simulink model "stanley_model"  (R2022a)
settings: Solver=FixedStepAuto  StartTime=0.0  StopTime=Ts  FixedStep=sampling  RelTol=1e-3
values from neighbouring files (symbols this model uses):
  curvature = (DX.*D2Y - DY.*D2X) ./(DX.^2+DY.^2).^(3/2)    [initiateHybrid.m]
  direction = ones(length(gradbp),1)    [initiateHybrid.m]
  gradbp = linspace(0,totalDistance,50)    [initiateHybrid.m]
  L = 3    [MultiAgent_initiateSAC.m]    (also in control_velocity.m; initiate.m; initiateHybrid.m; initiateSAC.m)
  ld = 5    [MultiAgent_initiateSAC.m]    (also in control_velocity.m; initiate.m; initiateHybrid.m; initiateSAC.m)
  psi_o = 0    [MultiAgent_initiateSAC.m]    (also in control_velocity.m; initiate.m; initiateHybrid.m = thetaRefs(1)*(pi/180); initiateSAC.m)
  thetaRefs = smooth(gradbp,thetaRef)    [initiateHybrid.m]
  vel = 5    [MultiAgent_initiateSAC.m]    (also in control_velocity.m = 7; initiate.m = 10; initiateHybrid.m; initiateSAC.m)
  X_o = refPose(1,1)+0    [MultiAgent_initiateSAC.m]    (also in control_velocity.m; initiate.m = refPose(1,1)+60; initiateHybrid.m = xRef(1); initiateSAC.m)
  xRef = refPose(:,1)    [MultiAgent_initiateSAC.m]    (also in control_velocity.m; initiate.m; initiateHybrid.m; initiateSAC.m)
  xRef2s = smooth(gradbp,xRef2)    [initiateHybrid.m]
  xteInt = sqrt((cnormal_xRef(idxc(1))-X_o)^2+(cnormal_yRef(idxc(1))-Y_o)^2)    [MultiAgent_initiateSAC.m]    (also in control_velocity.m; initiate.m; initiateSAC.m; initiateTD3.m)
  Y_o = -refPose(1,2)+20    [MultiAgent_initiateSAC.m]    (also in control_velocity.m = -refPose(1,2)+0; initiate.m; initiateHybrid.m = yRef(1); initiateSAC.m = -refPose(1,2)+0)
  yRef = -refPose(:,2)    [MultiAgent_initiateSAC.m]    (also in control_velocity.m; initiate.m; initiateHybrid.m; initiateSAC.m)
  yRef2s = smooth(gradbp,yRef2)    [initiateHybrid.m]
libraries: simulink_extras x2, simulink x2, vehdynlibviscommon x1, drivingvehiclecontroller x1, robotalgslib x1, autolibshared x1
settings Model: Creator=berka  LastModifiedBy=berka
settings DebuggingCC: UnconnectedInputMsg=warning  UnconnectedOutputMsg=warning  UnconnectedLineMsg=warning
settings RTWCC: DLArmComputeVersion=19.05

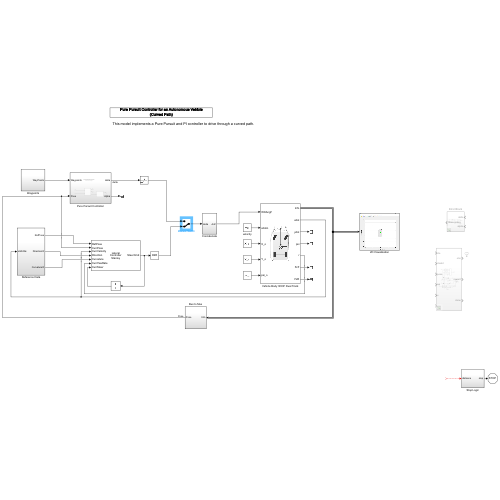
[thumbnail: Simulink's stored preview of the top-level diagram]
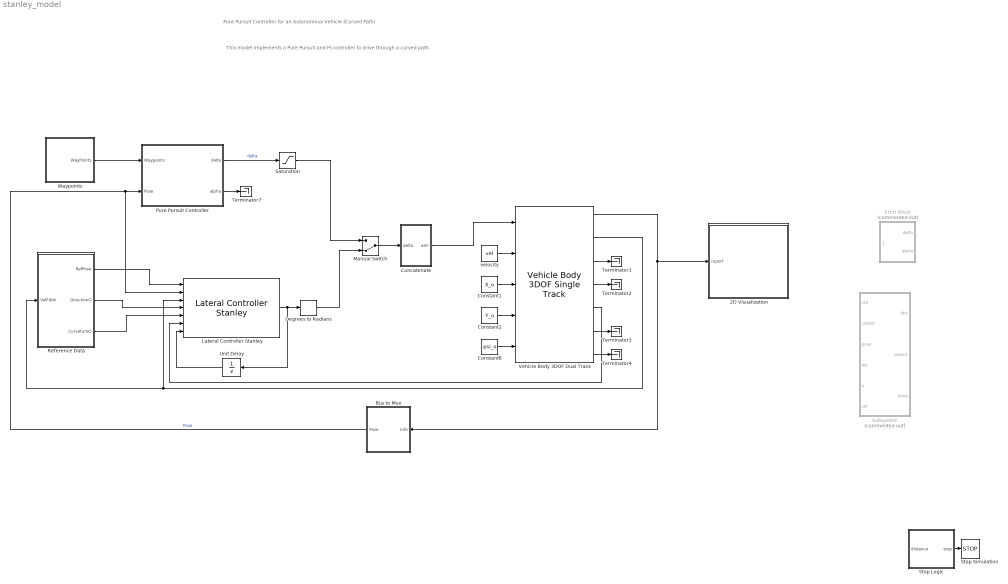
== system stanley_model ==
  note: This model implements a Pure Pursuit and PI controller to drive through a curved path.
  note: Pure Pursuit Controller for an Autonomous Vehicle
      | (Curved Path)
  2D Visualization : Subsystem
      mask Display: image("visualization.JPG");
  Bus to Mux : Subsystem
  Concatenate : Subsystem
  Constant1 : Constant  Value=X_o
  Constant2 : Constant  Value=Y_o
  Constant8 : Constant  Value=psi_o
  Degrees to Radians : simulink_extras/Transformations/Degrees to Radians
  Error Block : Subsystem  Commented=on
  Lateral Controller Stanley : drivingvehiclecontroller/Lateral Controller Stanley  ModelType=Dynamic bicycle model  PositionGainF=2.5  PositionGainR=2.5  YawRateGain=0.2  DelayGain=0.2  VehicleMass=2000  Lf=1.4  Lr=1.6  TireStiffness=12e3  Wheelbase=3  MaxSteeringAngle=35
      settings: SourceProductBaseCode=DR
  Manual Switch : ManualSwitch  CurrentSetting=0
  Pure Pursuit Controller : Subsystem
  Reference Data : Subsystem  VariantControl=Stanley
  Saturation : Saturate
  Stop Logic : Subsystem
  Stop Simulation : Stop
  Subsystem : Subsystem  Commented=on
  Terminator{1..4,7} (5 alike) : Terminator
  Unit Delay : UnitDelay  SampleTime=-1  HasFrameUpgradeWarning=on
  Vehicle Body 3DOF Dual Track : autolibshared/Vehicle Body 3DOF Single Track  trackMode=Dual  inputMode=External longitudinal velocity  frontSteerMode=on  rearSteerMode=off  windMode=off  muMode=off  extFMode=off  extMMode=off  htchFMode=off  htchMMode=off  extXo=on  extpsio=on  extxdoto=off  extro=off  extYo=on  extTamb=off  extydoto=off  aMode=2  NF=2  NR=2  m=2000  a=1.4  b=1.6  h=0.35  dh=1  hh=0.2  X_o=0  xdot_o=0  CalphaMode=off  sigmaMode=on  d=0  hl=0  w=[1.4,1.4]  Cy_f=12e3  Cy_r=11e3  sigma_f=.1  sigma_r=.1  alpha_f_brk=[-.1 .1]  Cy_f_data=[-9e3 9e3]  alpha_r_brk=[-.1 .1]  Cy_r_data=[-9e3 9e3]  Y_o=0  ydot_o=0  Izz=4000  psi_o=0  r_o=0  Af=2  Cd=.3  Cl=.1  Cpm=.1  beta_w=[0:0.01:0.3]  Cs=[0:0.03:0.9]  Cym=[0:0.01:0.3]  Pabs=101325  Tair=273  g=9.81  mu=1  xdot_tol=.01  Fznom=5000  Fxtire_sat=7e4  Fytire_sat=7e4  longOff=0  latOff=0  vertOff=0  wrapAng=off
      settings: SourceProductBaseCode=PW,DR,MT,VE
  Waypoints : Subsystem
  velocity : Constant  Value=vel
  wires:
  Constant1/1 -> Vehicle Body 3DOF Dual Track/3
  Vehicle Body 3DOF Dual Track/3 -> Terminator1/1
  Vehicle Body 3DOF Dual Track/1 -> Bus to Mux/1(Info), 2D Visualization/1(Inport)
  Constant8/1 -> Vehicle Body 3DOF Dual Track/5
  Concatenate/1(AnF) -> Vehicle Body 3DOF Dual Track/1
  Vehicle Body 3DOF Dual Track/6 -> Terminator3/1
  Constant2/1 -> Vehicle Body 3DOF Dual Track/4
  Vehicle Body 3DOF Dual Track/7 -> Terminator4/1
  Vehicle Body 3DOF Dual Track/4 -> Terminator2/1
  Vehicle Body 3DOF Dual Track/5 -> Lateral Controller Stanley/6
  Waypoints/1(WayPoints) -> Pure Pursuit Controller/1(Waypoints)
  Bus to Mux/1(Pose) -> Pure Pursuit Controller/2(Pose), Lateral Controller Stanley/2  "Pose"
  Pure Pursuit Controller/1(delta) -> Saturation/1  "delta"
  velocity/1 -> Vehicle Body 3DOF Dual Track/2
  Reference Data/2(DirectionO) -> Lateral Controller Stanley/4
  Reference Data/3(CurvatureO) -> Lateral Controller Stanley/5
  Reference Data/1(RefPose) -> Lateral Controller Stanley/1
  Lateral Controller Stanley/1 -> Unit Delay/1, Degrees to Radians/1
  Unit Delay/1 -> Lateral Controller Stanley/7
  ? -> Stop Logic/1(distance)
  Stop Logic/1(stop) -> Stop Simulation/1
  Pure Pursuit Controller/2(alpha) -> Terminator7/1
  Manual Switch/1 -> Concatenate/1(delta)
  Saturation/1 -> Manual Switch/1
  Degrees to Radians/1 -> Manual Switch/2
  Vehicle Body 3DOF Dual Track/2 -> Reference Data/1(VelFdbk), Lateral Controller Stanley/3

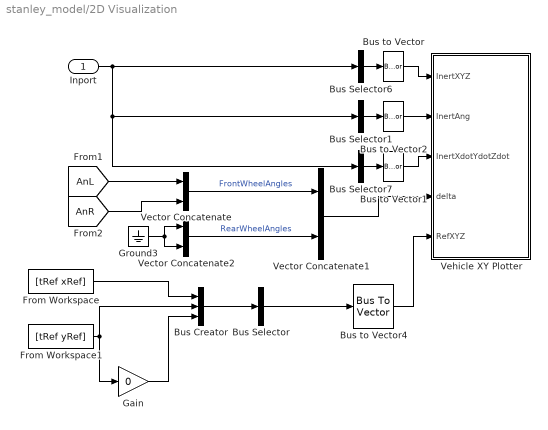
== system stanley_model/2D Visualization ==
  Inport : Inport
  Bus Creator : BusCreator  Inputs=3
  Bus Selector : BusSelector  OutputSignals=signal1,signal2,signal3  OutputAsBus=on
  Bus Selector1 : BusSelector  OutputSignals=InertFrm.Cg.Ang.phi,InertFrm.Cg.Ang.theta,InertFrm.Cg.Ang.psi  OutputAsBus=on
  Bus Selector6 : BusSelector  OutputSignals=InertFrm.Geom.Disp.X,InertFrm.Geom.Disp.Y,InertFrm.Geom.Disp.Z  OutputAsBus=on
  Bus Selector7 : BusSelector  OutputSignals=InertFrm.Geom.Vel.Xdot,InertFrm.Geom.Vel.Ydot,InertFrm.Geom.Vel.Zdot  OutputAsBus=on
  Bus to Vector{,1..2,4} (4 alike) : BusToVector
  From Workspace : FromWorkspace  VariableName=[tRef xRef]
  From Workspace1 : FromWorkspace  VariableName=[tRef yRef]
  Gain : Gain  Gain=0
  Ground3 : Ground
  Vector Concatenate : Concatenate
  Vector Concatenate1 : Concatenate
  Vector Concatenate2 : Concatenate
  Vehicle XY Plotter : Subsystem  mask(Vehicle XY Plotter){a=2, b=2, w=2, figBorder=10, bufferSize=1024, extRef=on, pltDT=.2}
      mask prompts: a "Distance to front axle from CG, a [m]:"; b "Distance to rear axle from CG, b [m]:"; w "Track width, w [m]:"; figBorder "Distance to figure borders, figBorder [m]:"; bufferSize "Path buffer sampe size, bufferSize []:"; extRef "Plot path reference, extRef"; pltDT "Plot update rate, pltDT [s]:"
      mask help:
      | This block will display a MATLAB figure which indicates the vehicle path, current position and heading velocity.
      | An optional path reference is also provided.
      mask init:
      | if autoblkschecksimstopped(gcb)
      |     PortName = 'RefXYZ';
      |     InportOption  = {'built-in/Ground', [PortName, ' Ground'];...
      |         'built-in/Inport',PortName };
      |     if ~strcmp(get_param(gcb,'extRef'),'on')
      |         NewBlkHdl = autoblksreplaceblock(gcb, InportOption, 1);
      |         set_param(NewBlkHdl, 'ShowName', 'off');
      |     else
      |         autoblksreplaceblock(gcb, InportOption, 2);
      |     end
      | end
      mask TypeOptions a: Vehicle XY Plotter/a
      mask TypeOptions b: Vehicle XY Plotter/b
      mask TypeOptions w: Vehicle XY Plotter/w
      mask TypeOptions figBorder: Vehicle XY Plotter/figBorder
      mask TypeOptions bufferSize: Vehicle XY Plotter/bufferSize
  wires:
  Vector Concatenate1/1 -> Vehicle XY Plotter/4(delta)
  Ground3/1 -> Vector Concatenate2/1, Vector Concatenate2/2
  Bus Selector6/1 -> Bus to Vector/1
  Vector Concatenate/1 -> Vector Concatenate1/1  "FrontWheelAngles"
  [AnL] -> Vector Concatenate/1
  Vector Concatenate2/1 -> Vector Concatenate1/2  "RearWheelAngles"
  Bus Selector7/1 -> Bus to Vector1/1
  Bus to Vector1/1 -> Vehicle XY Plotter/3(InertXdotYdotZdot)
  Bus to Vector/1 -> Vehicle XY Plotter/1(InertXYZ)
  Bus to Vector2/1 -> Vehicle XY Plotter/2(InertAng)
  Bus Selector1/1 -> Bus to Vector2/1
  [AnR] -> Vector Concatenate/2
  Inport/1 -> Bus Selector7/1, Bus Selector1/1, Bus Selector6/1
  Bus to Vector4/1 -> Vehicle XY Plotter/5(RefXYZ)
  Bus Selector/1 -> Bus to Vector4/1
  From Workspace1/1 -> Gain/1, Bus Creator/2
  Gain/1 -> Bus Creator/3
  From Workspace/1 -> Bus Creator/1
  Bus Creator/1 -> Bus Selector/1

== system stanley_model/Bus to Mux ==
  Info : Inport
  Bus Selector1 : BusSelector  OutputSignals=InertFrm.Cg.Disp.X,InertFrm.Cg.Disp.Y,InertFrm.Cg.Ang.psi
  Mux : Mux  Inputs=3
  Pose : Outport
  wires:
  Bus Selector1/3 -> Mux/3  "<psi>"
  Bus Selector1/1 -> Mux/1  "<X>"
  Mux/1 -> Pose/1
  Bus Selector1/2 -> Mux/2  "<Y>"
  Info/1 -> Bus Selector1/1

== system stanley_model/Concatenate ==
  delta : Inport
  Matrix Concatenate : Concatenate
  AnF : Outport  VectorParamsAs1DForOutWhenUnconnected=off
  tag scope: AnL=global, AnR=global
  wires:
  Matrix Concatenate/1 -> AnF/1
  delta/1 -> [AnL], [AnR], Matrix Concatenate/2, Matrix Concatenate/1

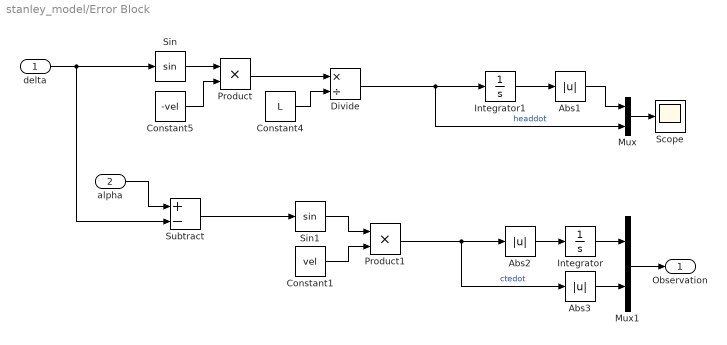
== system stanley_model/Error Block ==
  delta : Inport
  alpha : Inport  Port=2
  Abs1 : Abs  SaturateOnIntegerOverflow=off
  Abs2 : Abs  SaturateOnIntegerOverflow=off
  Abs3 : Abs  SaturateOnIntegerOverflow=off
  Constant1 : Constant  Value=vel
  Constant4 : Constant  Value=L
  Constant5 : Constant  Value=-vel
  Divide : Product  Inputs=*/
  Integrator : Integrator  InitialCondition=xteInt
  Integrator1 : Integrator
  Mux : Mux  Inputs=2
  Mux1 : Mux  Inputs=2
  Product : Product
  Product1 : Product
  Scope : Scope
  Sin : Trigonometry
  Sin1 : Trigonometry
  Subtract : Sum  Inputs=+-
  Observation : Outport
  wires:
  Constant4/1 -> Divide/2
  Sin/1 -> Product/1
  Product/1 -> Divide/1
  delta/1 -> Subtract/2, Sin/1
  Constant5/1 -> Product/2
  Sin1/1 -> Product1/1
  Constant1/1 -> Product1/2
  Subtract/1 -> Sin1/1
  alpha/1 -> Subtract/1
  Divide/1 -> Integrator1/1, Mux/2  "headdot"
  Product1/1 -> Abs3/1, Abs2/1  "ctedot"
  Integrator1/1 -> Abs1/1
  Abs1/1 -> Mux/1
  Mux/1 -> Scope/1
  Mux1/1 -> Observation/1
  Integrator/1 -> Mux1/1
  Abs3/1 -> Mux1/2
  Abs2/1 -> Integrator/1

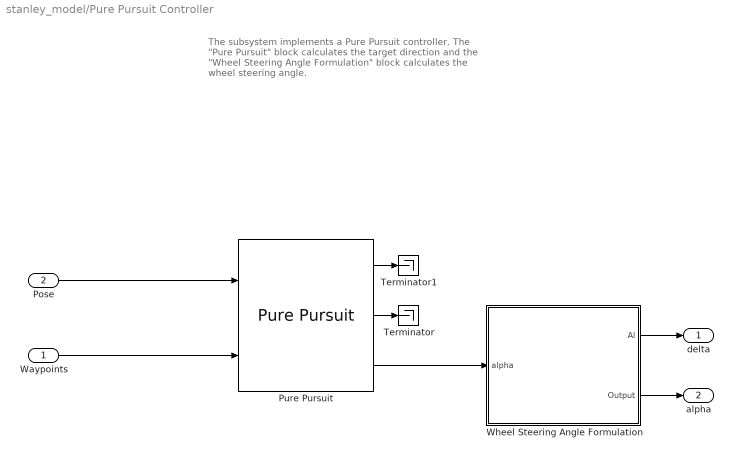
== system stanley_model/Pure Pursuit Controller ==
  note: The subsystem implements a Pure Pursuit controller. The "Pure Pursuit" block calculates the target direction and the "Wheel Steering Angle Formulation" block calculates the wheel steering angle.
  Waypoints : Inport
  Pose : Inport  Port=2
  Pure Pursuit : robotalgslib/Pure Pursuit  DesiredLinearVelocity=4.1102  MaxAngularVelocity=1.0  LookaheadDistance=2.6305  TargetDirPort=on  SimulateUsing=Code generation
  Terminator : Terminator
  Terminator1 : Terminator
  Wheel Steering Angle Formulation : Subsystem  mask{L=L, ld=ld}
      mask prompts: L "Bicycle length"; ld "Lookahead distance"
      mask TypeOptions L: Bicycle length/Value
      mask TypeOptions ld: Lookahead distance/Value
      mask Display:
      | image("GeometryMask.png")
      | port_label('input', 1, 'alpha')
      | port_label('output', 1, 'delta')
  delta : Outport
  alpha : Outport  Port=2
  wires:
  Pure Pursuit/3 -> Wheel Steering Angle Formulation/1(alpha)
  Waypoints/1 -> Pure Pursuit/2
  Pose/1 -> Pure Pursuit/1
  Pure Pursuit/1 -> Terminator1/1
  Pure Pursuit/2 -> Terminator/1
  Wheel Steering Angle Formulation/1(Al) -> delta/1
  Wheel Steering Angle Formulation/2(Output) -> alpha/1

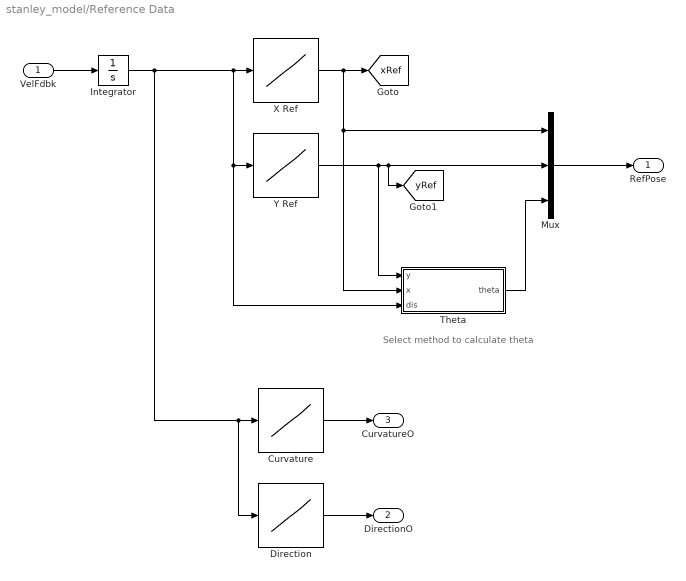
== system stanley_model/Reference Data ==
  note: Select method to calculate theta
  VelFdbk : Inport
  Curvature : Lookup_n-D  NumberOfTableDimensions=1  BreakpointsForDimension1=gradbp  Table=curvature  InternalRulePriority=Speed  RndMeth=Simplest
  Direction : Lookup_n-D  NumberOfTableDimensions=1  BreakpointsForDimension1=gradbp  Table=direction  InternalRulePriority=Speed  RndMeth=Simplest
  Integrator : Integrator
  Mux : Mux  Inputs=3
  Theta : Subsystem  Variant=on  VariantControlMode=label  LabelModeActiveChoice=thetaSimulinkBlock
  X Ref : Lookup_n-D  NumberOfTableDimensions=1  BreakpointsForDimension1=gradbp  Table=xRef2s  InternalRulePriority=Speed  RndMeth=Simplest
  Y Ref : Lookup_n-D  NumberOfTableDimensions=1  BreakpointsForDimension1=gradbp  Table=yRef2s  InternalRulePriority=Speed  RndMeth=Simplest
  RefPose : Outport
  DirectionO : Outport  Port=2
  CurvatureO : Outport  Port=3
  tag scope: xRef=global, yRef=global
  wires:
  Direction/1 -> DirectionO/1
  Curvature/1 -> CurvatureO/1
  Y Ref/1 -> Theta/1(y), Mux/2, [yRef]
  Mux/1 -> RefPose/1
  X Ref/1 -> Theta/2(x), Mux/1, [xRef]
  Integrator/1 -> Curvature/1, Direction/1, Theta/3(dis), Y Ref/1, X Ref/1
  VelFdbk/1 -> Integrator/1
  Theta/1(theta) -> Mux/3

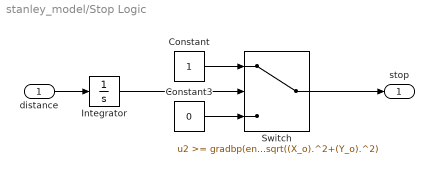
== system stanley_model/Stop Logic ==
  distance : Inport
  Constant : Constant
  Constant3 : Constant  Value=0
  Integrator : Integrator  InitialCondition=sqrt((X_o).^2+(Y_o).^2)
  Switch : Switch  Threshold=gradbp(end)+sqrt((X_o).^2+(Y_o).^2)  SaturateOnIntegerOverflow=off  InputSameDT=off
  stop : Outport
  wires:
  Switch/1 -> stop/1
  Constant3/1 -> Switch/3
  distance/1 -> Integrator/1
  Constant/1 -> Switch/1
  Integrator/1 -> Switch/2

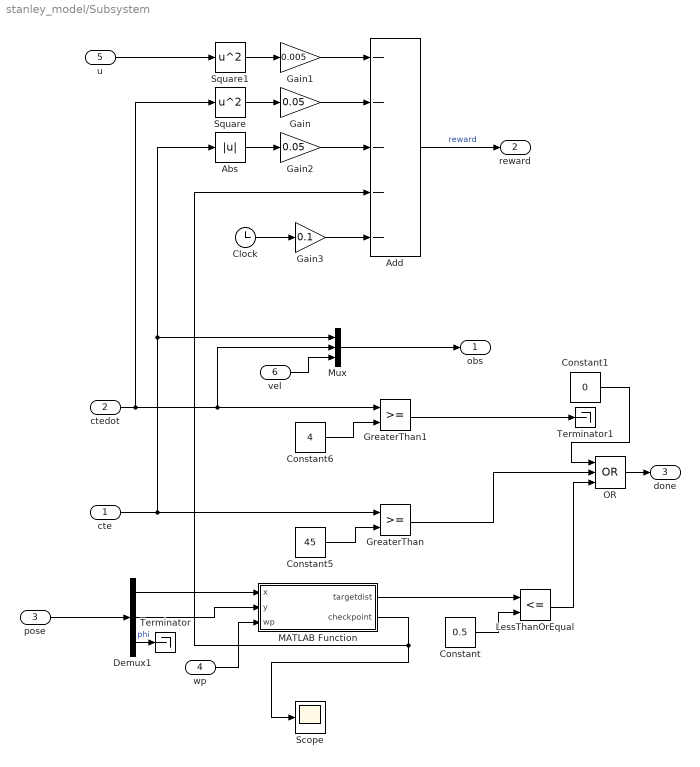
== system stanley_model/Subsystem ==
  cte : Inport
  ctedot : Inport  Port=2
  pose : Inport  Port=3
  wp : Inport  Port=4
  u : Inport  Port=5
  vel : Inport  Port=6
  Abs : Abs  SaturateOnIntegerOverflow=off
  Add : Sum  Inputs=-----
  Clock : Clock
  Constant : Constant  Value=0.5
  Constant1 : Constant  Value=0
  Constant5 : Constant  Value=45
  Constant6 : Constant  Value=4
  Demux1 : Demux  Outputs=3
  Gain : Gain  Gain=0.05
  Gain1 : Gain  Gain=0.005
  Gain2 : Gain  Gain=0.05
  Gain3 : Gain  Gain=0.1
  GreaterThan : RelationalOperator  OutDataTypeStr=boolean  RndMeth=Simplest  InputSameDT=off
  GreaterThan1 : RelationalOperator  OutDataTypeStr=boolean  RndMeth=Simplest  InputSameDT=off
  LessThanOrEqual : RelationalOperator  Operator=<=  OutDataTypeStr=boolean  RndMeth=Simplest  InputSameDT=off
  MATLAB Function : MATLAB Function  TreatAsAtomicUnit=on
  Mux : Mux  Inputs=3
  OR : Logic  Operator=OR  Inputs=3  IconShape=distinctive  AllPortsSameDT=off  OutDataTypeStr=boolean
  Scope : Scope
  Square : Math  Operator=square
  Square1 : Math  Operator=square
  Terminator : Terminator
  Terminator1 : Terminator
  obs : Outport
  reward : Outport  Port=2
  done : Outport  Port=3
  wires:
  Constant5/1 -> GreaterThan/2
  Constant6/1 -> GreaterThan1/2
  GreaterThan/1 -> OR/2
  GreaterThan1/1 -> Terminator1/1
  Mux/1 -> obs/1
  Constant/1 -> LessThanOrEqual/2
  Demux1/2 -> MATLAB Function/2(y)
  Demux1/1 -> MATLAB Function/1(x)
  MATLAB Function/1(targetdist) -> LessThanOrEqual/1
  pose/1 -> Demux1/1
  Demux1/3 -> Terminator/1  "phi"
  wp/1 -> MATLAB Function/3(wp)
  cte/1 -> Mux/1, Abs/1, GreaterThan/1
  Abs/1 -> Gain2/1
  Square1/1 -> Gain1/1
  Gain/1 -> Add/2
  Gain1/1 -> Add/1
  ctedot/1 -> Square/1, GreaterThan1/1, Mux/2
  Square/1 -> Gain/1
  u/1 -> Square1/1
  Add/1 -> reward/1  "reward"
  Gain2/1 -> Add/3
  MATLAB Function/2(checkpoint) -> Scope/1, Add/4
  OR/1 -> done/1
  LessThanOrEqual/1 -> OR/3
  Constant1/1 -> OR/1
  vel/1 -> Mux/3
  Gain3/1 -> Add/5
  Clock/1 -> Gain3/1

== system stanley_model/Waypoints ==
  Constant3 : Constant  Value=xRef  SampleTime=0.1
  Constant4 : Constant  Value=yRef  SampleTime=0.1
  Matrix Concatenate : Concatenate  Mode=Multidimensional array  ConcatenateDimension=2
  WayPoints : Outport
  wires:
  Constant4/1 -> Matrix Concatenate/2
  Matrix Concatenate/1 -> WayPoints/1
  Constant3/1 -> Matrix Concatenate/1

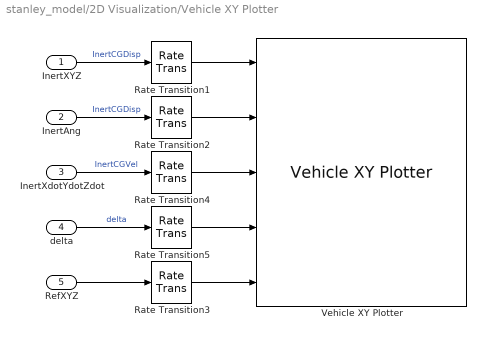
== system stanley_model/2D Visualization/Vehicle XY Plotter ==
  InertXYZ : Inport
  InertAng : Inport  Port=2
  InertXdotYdotZdot : Inport  Port=3
  delta : Inport  Port=4
  RefXYZ : Inport  Port=5
  Rate Transition{1..5} (5 alike) : RateTransition  Deterministic=off  OutPortSampleTime=pltDT
  Vehicle XY Plotter : vehdynlibviscommon/Vehicle XY Plotter  w=w  a=a  b=b  figBorder=figBorder  bufferSize=bufferSize  extStats=off  extTireF=off
      settings: SourceProductBaseCode=VE
  wires:
  Rate Transition5/1 -> Vehicle XY Plotter/4
  Rate Transition4/1 -> Vehicle XY Plotter/3
  Rate Transition2/1 -> Vehicle XY Plotter/2
  Rate Transition1/1 -> Vehicle XY Plotter/1
  Rate Transition3/1 -> Vehicle XY Plotter/5
  delta/1 -> Rate Transition5/1  "delta"
  InertXYZ/1 -> Rate Transition1/1  "InertCGDisp"
  InertXdotYdotZdot/1 -> Rate Transition4/1  "InertCGVel"
  InertAng/1 -> Rate Transition2/1  "InertCGDisp"
  RefXYZ/1 -> Rate Transition3/1

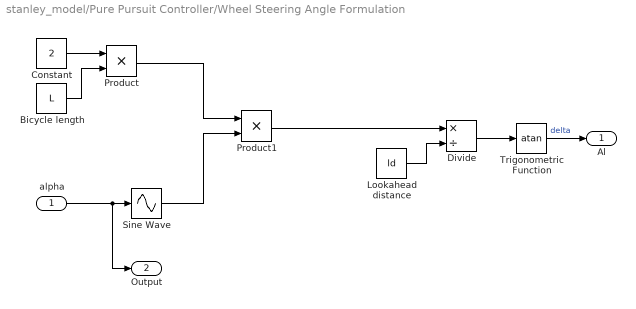
== system stanley_model/Pure Pursuit Controller/Wheel Steering Angle Formulation ==
  alpha : Inport
  Bicycle length : Constant  Value=L
  Constant : Constant  Value=2
  Divide : Product  Inputs=*/
  Lookahead distance : Constant  Value=ld
  Product : Product
  Product1 : Product
  Sine Wave : Sin  TimeSource=Use external signal  SampleTime=0
  Trigonometric Function : Trigonometry  Operator=atan
  Al : Outport
  Output : Outport  Port=2
  wires:
  Sine Wave/1 -> Product1/2
  Bicycle length/1 -> Product/2
  Constant/1 -> Product/1
  Product1/1 -> Divide/1
  Product/1 -> Product1/1
  Divide/1 -> Trigonometric Function/1
  Trigonometric Function/1 -> Al/1  "delta"
  alpha/1 -> Output/1, Sine Wave/1
  Lookahead distance/1 -> Divide/2

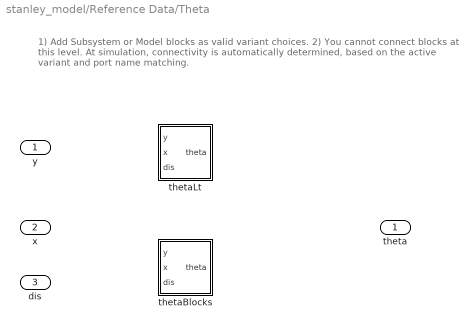
== system stanley_model/Reference Data/Theta ==
  note: 1) Add Subsystem or Model blocks as valid variant choices.
      | 2) You cannot connect blocks at this level. At simulation, connectivity is automatically
      | determined, based on the active variant and port name matching.
  y : Inport
  x : Inport  Port=2
  dis : Inport  Port=3
  thetaBlocks : Subsystem  VariantControl=thetaSimulinkBlock
  thetaLt : Subsystem  VariantControl=thetaLookUpTable
  theta : Outport

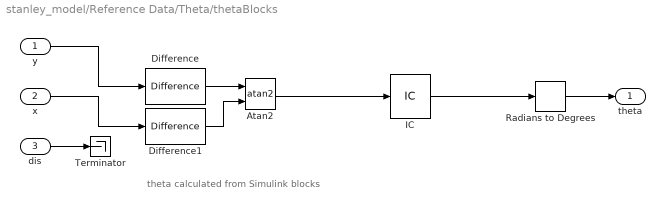
== system stanley_model/Reference Data/Theta/thetaBlocks ==
  note: theta calculated from Simulink blocks
  y : Inport
  x : Inport  Port=2
  dis : Inport  Port=3
  Atan2 : Trigonometry  Operator=atan2  ApproximationMethod=CORDIC
  Difference : simulink/Discrete/Difference  ICPrevInput=0.0  OutMin=[]  OutMax=[]  OutDataType=fixdt(1, 16)  OutScaling=2^-10  DoSatur=off
  Difference1 : simulink/Discrete/Difference  ICPrevInput=0.0  OutMin=[]  OutMax=[]  OutDataType=fixdt(1, 16)  OutScaling=2^-10  DoSatur=off
  IC : InitialCondition  Value=psi_o
  Radians to Degrees : simulink_extras/Transformations/Radians to Degrees
  Terminator : Terminator
  theta : Outport
  wires:
  IC/1 -> Radians to Degrees/1
  Atan2/1 -> IC/1
  dis/1 -> Terminator/1
  x/1 -> Difference1/1
  y/1 -> Difference/1
  Radians to Degrees/1 -> theta/1
  Difference/1 -> Atan2/1
  Difference1/1 -> Atan2/2

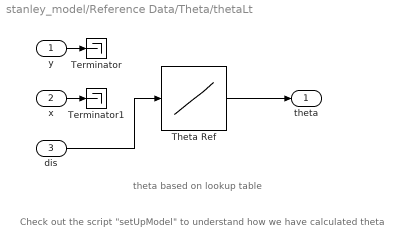
== system stanley_model/Reference Data/Theta/thetaLt ==
  note: Check out the script "setUpModel" to understand how we have calculated theta
  note: theta based on lookup table
  y : Inport
  x : Inport  Port=2
  dis : Inport  Port=3
  Terminator : Terminator
  Terminator1 : Terminator
  Theta Ref : Lookup_n-D  NumberOfTableDimensions=1  BreakpointsForDimension1=gradbp  Table=thetaRefs  InternalRulePriority=Speed  RndMeth=Simplest
  theta : Outport
  wires:
  Theta Ref/1 -> theta/1
  dis/1 -> Theta Ref/1
  x/1 -> Terminator1/1
  y/1 -> Terminator/1

== matlab function stanley_model/Subsystem/MATLAB Function ==
  data: x input; targetdist output; y input; wp input; checkpoint output
function [targetdist, checkpoint] = fcn(x,y,wp)

x_last = wp(end,1);
y_last = wp(end,2);
targetdist = sqrt((x_last-x)^2 + (y_last-y)^2);

checkpoint = 0;

end
